simulink library "pathProjection_ul"  (R2018a)
settings: Solver=VariableStepAuto  StartTime=0.0  StopTime=10.0  RelTol=1e-3
values from neighbouring files (symbols this model uses):
  searchDistance_none = 0.2    [pathProjection_init.m]
undefined symbols (not defined in the file or in its folder): pathHeight_m, pathWidth_m
settings Model: Creator=mcobb  LastModifiedBy=mcobb

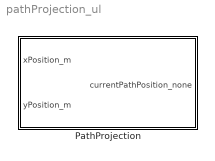
== system pathProjection_ul ==
  PathProjection : Subsystem

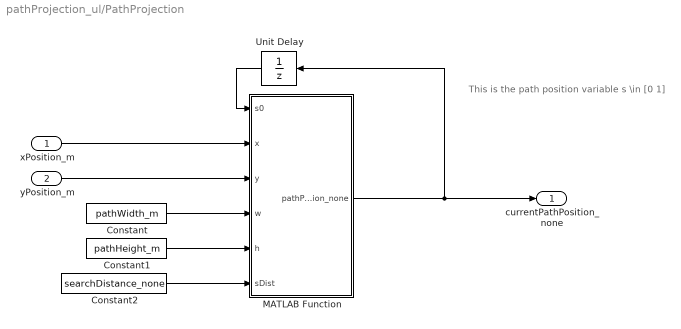
== system pathProjection_ul/PathProjection ==
  note: This is the path position variable s \in [0 1]
  xPosition_m : Inport
  yPosition_m : Inport  Port=2
  Constant : Constant  Value=pathWidth_m
  Constant1 : Constant  Value=pathHeight_m
  Constant2 : Constant  Value=searchDistance_none
  MATLAB Function : MATLAB Function  TreatAsAtomicUnit=on
  Unit Delay : UnitDelay  SampleTime=-1
  currentPathPosition_none : Outport
  wires:
  Unit Delay/1 -> MATLAB Function/1(s0)
  xPosition_m/1 -> MATLAB Function/2(x)
  yPosition_m/1 -> MATLAB Function/3(y)
  Constant/1 -> MATLAB Function/4(w)
  Constant1/1 -> MATLAB Function/5(h)
  Constant2/1 -> MATLAB Function/6(sDist)
  MATLAB Function/1(pathPosition_none) -> Unit Delay/1, currentPathPosition_none/1

== matlab function pathProjection_ul/PathProjection/MATLAB Function ==
  data: s0 input; pathPosition_none output; x input; y input; w input; h input; sDist input
function pathPosition_none = fcn(s0,x,y,w,h,sDist)
pathPosition_none = pathProjection(s0,x,y,w,h,sDist);
end
